simulink model "UberSpurs"  (R2015b)
settings: Solver=VariableStepAuto  StartTime=0.0  StopTime=5000  RelTol=1e-3
libraries: simulink x54
(part 2 of 6)

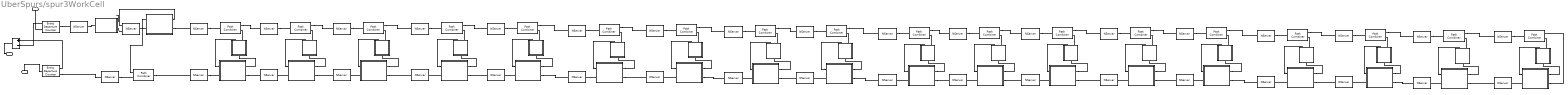
== system UberSpurs/spur3WorkCell ==
  Add1 : Sum  Inputs=+-
  INFlowCount : EntityDepartureCounter  NumberDepartedToSignal=on  NumberDepartedToAttribute=off
  OUTFlowCount : EntityDepartureCounter  NumberDepartedToSignal=on  NumberDepartedToAttribute=off
  combineRecirculate : PathCombiner  NumberInputPorts=2
  fillChannel1 : Subsystem
  fillChannel10 : Subsystem
  fillChannel11 : Subsystem
  fillChannel12 : Subsystem
  fillChannel13 : Subsystem
  fillChannel14 : Subsystem
  fillChannel15 : Subsystem
  fillChannel16 : Subsystem
  fillChannel17 : Subsystem
  fillChannel18 : Subsystem
  fillChannel2 : Subsystem
  fillChannel3 : Subsystem
  fillChannel4 : Subsystem
  fillChannel5 : Subsystem
  fillChannel6 : Subsystem
  fillChannel7 : Subsystem
  fillChannel8 : Subsystem
  fillChannel9 : Subsystem
  fromChannel{1..18} (18 alike) : PathCombiner  NumberInputPorts=2
  route2Channel1 : Subsystem
  route2Channel10 : Subsystem
  route2Channel11 : Subsystem
  route2Channel12 : Subsystem
  route2Channel13 : Subsystem
  route2Channel14 : Subsystem
  route2Channel15 : Subsystem
  route2Channel16 : Subsystem
  route2Channel17 : Subsystem
  route2Channel18 : Subsystem
  route2Channel2 : Subsystem
  route2Channel3 : Subsystem
  route2Channel4 : Subsystem
  route2Channel5 : Subsystem
  route2Channel6 : Subsystem
  route2Channel7 : Subsystem
  route2Channel8 : Subsystem
  route2Channel9 : Subsystem
  route2recirculate : Subsystem
  toChannel : NServer  NumberOfServers=15  ServiceTime=6
  toChannel{1..18} (18 alike) : NServer  NumberOfServers=2  ServiceTime=0.8
  toMainConveyor : NServer  ServiceTime=2
  toRecirculate : NServer  NumberOfServers=3
  toVerify : NServer  NumberOfServers=12  ServiceTime=5  StatNumberInBlock=on
      settings: OutputPortMap=o1
  toVerify{1..17} (17 alike) : NServer  NumberOfServers=2  ServiceTime=0.8
  verifyWorkstation : Subsystem
  toMHS : PMIOPort  Port=1  Side=Left
  fromMHS : PMIOPort  Port=2  Side=Left
  WIP : Outport
  wires:
  fillChannel1/1(serverAvailable) -> route2Channel1/1(serverAvailable)
  INFlowCount/1 -> Add1/1
  OUTFlowCount/1 -> Add1/2
  Add1/1 -> WIP/1
  fillChannel2/1(serverAvailable) -> route2Channel2/1(serverAvailable)
  fillChannel3/1(serverAvailable) -> route2Channel3/1(serverAvailable)
  fillChannel4/1(serverAvailable) -> route2Channel4/1(serverAvailable)
  fillChannel5/1(serverAvailable) -> route2Channel5/1(serverAvailable)
  fillChannel6/1(serverAvailable) -> route2Channel6/1(serverAvailable)
  fillChannel7/1(serverAvailable) -> route2Channel7/1(serverAvailable)
  fillChannel8/1(serverAvailable) -> route2Channel8/1(serverAvailable)
  fillChannel9/1(serverAvailable) -> route2Channel9/1(serverAvailable)
  fillChannel10/1(serverAvailable) -> route2Channel10/1(serverAvailable)
  fillChannel11/1(serverAvailable) -> route2Channel11/1(serverAvailable)
  fillChannel12/1(serverAvailable) -> route2Channel12/1(serverAvailable)
  fillChannel13/1(serverAvailable) -> route2Channel13/1(serverAvailable)
  fillChannel14/1(serverAvailable) -> route2Channel14/1(serverAvailable)
  fillChannel15/1(serverAvailable) -> route2Channel15/1(serverAvailable)
  fillChannel16/1(serverAvailable) -> route2Channel16/1(serverAvailable)
  fillChannel17/1(serverAvailable) -> route2Channel17/1(serverAvailable)
  fillChannel18/1(serverAvailable) -> route2Channel18/1(serverAvailable)
  toVerify/1 -> route2recirculate/1(verifyQueueLength)
  verifyWorkstation/1(queueLength) -> ?
  connections:
  fillChannel1/LConn1 -- route2Channel1/RConn1
  toChannel1/RConn1 -- route2Channel1/LConn1
  combineRecirculate/RConn1 -- toChannel1/LConn1
  route2recirculate/RConn1 -- combineRecirculate/LConn1
  OUTFlowCount/RConn1 -- toMHS/RConn1
  fromMHS/RConn1 -- INFlowCount/LConn1
  fillChannel1/RConn1 -- fromChannel1/LConn2
  toRecirculate/LConn1 -- fromChannel1/RConn1
  route2recirculate/LConn1 -- toRecirculate/RConn1
  route2Channel2/RConn1 -- fillChannel2/LConn1
  fillChannel2/RConn1 -- fromChannel2/LConn2
  route2Channel2/LConn1 -- toChannel2/RConn1
  toVerify1/LConn1 -- fromChannel2/RConn1
  route2Channel3/RConn1 -- fillChannel3/LConn1
  fillChannel3/RConn1 -- fromChannel3/LConn2
  route2Channel3/LConn1 -- toChannel3/RConn1
  toVerify2/LConn1 -- fromChannel3/RConn1
  route2Channel4/RConn1 -- fillChannel4/LConn1
  fillChannel4/RConn1 -- fromChannel4/LConn2
  route2Channel4/LConn1 -- toChannel4/RConn1
  toVerify3/LConn1 -- fromChannel4/RConn1
  route2Channel5/RConn1 -- fillChannel5/LConn1
  fillChannel5/RConn1 -- fromChannel5/LConn2
  route2Channel5/LConn1 -- toChannel5/RConn1
  toVerify4/LConn1 -- fromChannel5/RConn1
  route2Channel6/RConn1 -- fillChannel6/LConn1
  fillChannel6/RConn1 -- fromChannel6/LConn2
  route2Channel6/LConn1 -- toChannel6/RConn1
  toVerify5/LConn1 -- fromChannel6/RConn1
  route2Channel7/RConn1 -- fillChannel7/LConn1
  fillChannel7/RConn1 -- fromChannel7/LConn2
  route2Channel7/LConn1 -- toChannel7/RConn1
  toVerify6/LConn1 -- fromChannel7/RConn1
  route2Channel8/RConn1 -- fillChannel8/LConn1
  fillChannel8/RConn1 -- fromChannel8/LConn2
  route2Channel8/LConn1 -- toChannel8/RConn1
  toVerify7/LConn1 -- fromChannel8/RConn1
  route2Channel9/RConn1 -- fillChannel9/LConn1
  fillChannel9/RConn1 -- fromChannel9/LConn2
  route2Channel9/LConn1 -- toChannel9/RConn1
  toVerify8/LConn1 -- fromChannel9/RConn1
  fromChannel1/LConn1 -- toVerify1/RConn1
  route2Channel1/RConn2 -- toChannel2/LConn1
  route2Channel2/RConn2 -- toChannel3/LConn1
  fromChannel2/LConn1 -- toVerify2/RConn1
  fromChannel3/LConn1 -- toVerify3/RConn1
  route2Channel3/RConn2 -- toChannel4/LConn1
  fromChannel4/LConn1 -- toVerify4/RConn1
  route2Channel4/RConn2 -- toChannel5/LConn1
  fromChannel5/LConn1 -- toVerify5/RConn1
  route2Channel5/RConn2 -- toChannel6/LConn1
  fromChannel6/LConn1 -- toVerify6/RConn1
  route2Channel6/RConn2 -- toChannel7/LConn1
  fromChannel7/LConn1 -- toVerify7/RConn1
  route2Channel7/RConn2 -- toChannel8/LConn1
  fromChannel8/LConn1 -- toVerify8/RConn1
  route2Channel8/RConn2 -- toChannel9/LConn1
  route2Channel10/RConn2 -- toChannel11/LConn1
  route2Channel12/LConn1 -- toChannel12/RConn1
  route2Channel18/RConn1 -- fillChannel18/LConn1
  fromChannel17/LConn1 -- toVerify17/RConn1
  route2Channel13/RConn2 -- toChannel14/LConn1
  toVerify11/LConn1 -- fromChannel12/RConn1
  fillChannel10/RConn1 -- fromChannel10/LConn2
  fillChannel16/RConn1 -- fromChannel16/LConn2
  toVerify15/LConn1 -- fromChannel16/RConn1
  fromChannel14/LConn1 -- toVerify14/RConn1
  fillChannel15/RConn1 -- fromChannel15/LConn2
  toVerify14/LConn1 -- fromChannel15/RConn1
  route2Channel17/RConn2 -- toChannel18/LConn1
  fromChannel10/LConn1 -- toVerify10/RConn1
  toVerify17/LConn1 -- fromChannel18/RConn1
  route2Channel15/RConn2 -- toChannel16/LConn1
  route2Channel16/LConn1 -- toChannel16/RConn1
  route2Channel11/RConn2 -- toChannel12/LConn1
  toVerify9/LConn1 -- fromChannel10/RConn1
  route2Channel16/RConn2 -- toChannel17/LConn1
  fromChannel15/LConn1 -- toVerify15/RConn1
  toVerify12/LConn1 -- fromChannel13/RConn1
  route2Channel16/RConn1 -- fillChannel16/LConn1
  fromChannel13/LConn1 -- toVerify13/RConn1
  route2Channel15/RConn1 -- fillChannel15/LConn1
  fromChannel16/LConn1 -- toVerify16/RConn1
  route2Channel12/RConn1 -- fillChannel12/LConn1
  fillChannel18/RConn1 -- fromChannel18/LConn2
  route2Channel15/LConn1 -- toChannel15/RConn1
  route2Channel12/RConn2 -- toChannel13/LConn1
  route2Channel18/LConn1 -- toChannel18/RConn1
  fillChannel12/RConn1 -- fromChannel12/LConn2
  route2Channel14/RConn2 -- toChannel15/LConn1
  fromChannel11/LConn1 -- toVerify11/RConn1
  fromChannel12/LConn1 -- toVerify12/RConn1
  route2Channel13/LConn1 -- toChannel13/RConn1
  route2Channel10/LConn1 -- toChannel10/RConn1
  toVerify13/LConn1 -- fromChannel14/RConn1
  route2Channel17/RConn1 -- fillChannel17/LConn1
  fillChannel14/RConn1 -- fromChannel14/LConn2
  fillChannel11/RConn1 -- fromChannel11/LConn2
  route2Channel10/RConn1 -- fillChannel10/LConn1
  route2Channel11/LConn1 -- toChannel11/RConn1
  fillChannel17/RConn1 -- fromChannel17/LConn2
  route2Channel17/LConn1 -- toChannel17/RConn1
  route2Channel14/LConn1 -- toChannel14/RConn1
  toVerify16/LConn1 -- fromChannel17/RConn1
  route2Channel13/RConn1 -- fillChannel13/LConn1
  fillChannel13/RConn1 -- fromChannel13/LConn2
  route2Channel14/RConn1 -- fillChannel14/LConn1
  route2Channel11/RConn1 -- fillChannel11/LConn1
  toVerify10/LConn1 -- fromChannel11/RConn1
  fromChannel9/LConn1 -- toVerify9/RConn1
  route2Channel9/RConn2 -- toChannel10/LConn1
  route2Channel18/RConn2 -- fromChannel18/LConn1
  toChannel/RConn1 -- combineRecirculate/LConn2
  INFlowCount/RConn1 -- toChannel/LConn1
  toVerify/RConn1 -- verifyWorkstation/RConn1
  toVerify/LConn1 -- route2recirculate/RConn2
  toMainConveyor/LConn1 -- verifyWorkstation/LConn1
  OUTFlowCount/LConn1 -- toMainConveyor/RConn1

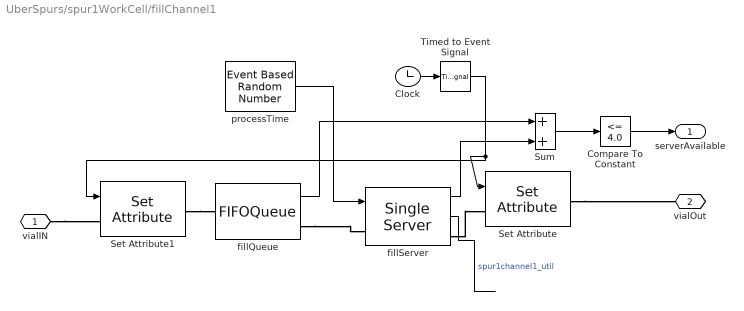
== system UberSpurs/spur1WorkCell/fillChannel1 ==
  Clock : Clock
  Compare To Constant : simulink/Logic and Bit Operations/Compare To Constant  relop=<=  const=4.0  OutDataTypeStr=boolean
  Set Attribute : SetAttribute  AttributeName=FillTime  AttributeFrom=Signal port  EvaluatedAttributeValue={ []}
  Set Attribute1 : SetAttribute  AttributeName=FillTimeIN  AttributeFrom=Signal port  EvaluatedAttributeValue={ []}
  Sum : Sum  Inputs=|++
  Timed to Event Signal : TimedToEventSignal
  fillQueue : FIFOQueue  Capacity=3  StatNumberInBlock=on
      settings: OutputPortMap=o1
  fillServer : SingleServer  ServiceTimeFrom=Signal port t  ServiceTime=20  StatNumberInBlock=on  StatUtilization=on
      settings: OutputPortMap=o1,o5
  processTime : EventBasedRandomNumber  Distribution=Gaussian (normal)  meanNorm=12  stdNorm=0.6  Seed=31208
  vialIN : PMIOPort  Port=1  Side=Left
  vialOut : PMIOPort  Port=2  Side=Right
  serverAvailable : Outport
  wires:
  processTime/1 -> fillServer/1
  Clock/1 -> Timed to Event Signal/1
  Timed to Event Signal/1 -> Set Attribute1/1, Set Attribute/1
  fillQueue/1 -> Sum/1
  fillServer/1 -> Sum/2
  Sum/1 -> Compare To Constant/1
  Compare To Constant/1 -> serverAvailable/1
  fillServer/2 -> ?  "spur1channel1_util"
  connections:
  fillQueue/RConn1 -- fillServer/LConn1
  fillServer/RConn1 -- Set Attribute/LConn1
  Set Attribute/RConn1 -- vialOut/RConn1
  vialIN/RConn1 -- Set Attribute1/LConn1
  Set Attribute1/RConn1 -- fillQueue/LConn1

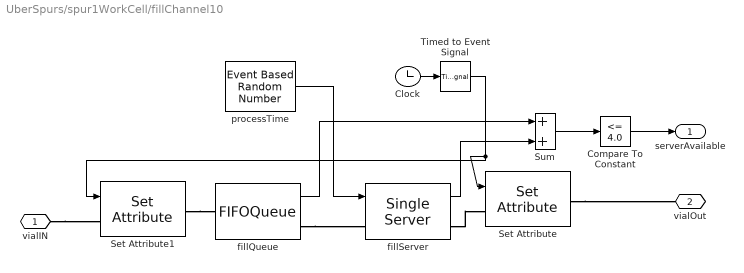
== system UberSpurs/spur1WorkCell/fillChannel10 ==
  Clock : Clock
  Compare To Constant : simulink/Logic and Bit Operations/Compare To Constant  relop=<=  const=4.0  OutDataTypeStr=boolean
  Set Attribute : SetAttribute  AttributeName=FillTime  AttributeFrom=Signal port  EvaluatedAttributeValue={ []}
  Set Attribute1 : SetAttribute  AttributeName=FillTimeIN  AttributeFrom=Signal port  EvaluatedAttributeValue={ []}
  Sum : Sum  Inputs=|++
  Timed to Event Signal : TimedToEventSignal
  fillQueue : FIFOQueue  Capacity=3  StatNumberInBlock=on
      settings: OutputPortMap=o1
  fillServer : SingleServer  ServiceTimeFrom=Signal port t  ServiceTime=20  StatNumberInBlock=on
      settings: OutputPortMap=o1
  processTime : EventBasedRandomNumber  Distribution=Gaussian (normal)  meanNorm=12  stdNorm=0.6  Seed=34425
  vialIN : PMIOPort  Port=1  Side=Left
  vialOut : PMIOPort  Port=2  Side=Right
  serverAvailable : Outport
  wires:
  processTime/1 -> fillServer/1
  Clock/1 -> Timed to Event Signal/1
  Timed to Event Signal/1 -> Set Attribute1/1, Set Attribute/1
  fillQueue/1 -> Sum/1
  fillServer/1 -> Sum/2
  Sum/1 -> Compare To Constant/1
  Compare To Constant/1 -> serverAvailable/1
  connections:
  fillQueue/RConn1 -- fillServer/LConn1
  fillServer/RConn1 -- Set Attribute/LConn1
  Set Attribute/RConn1 -- vialOut/RConn1
  vialIN/RConn1 -- Set Attribute1/LConn1
  Set Attribute1/RConn1 -- fillQueue/LConn1

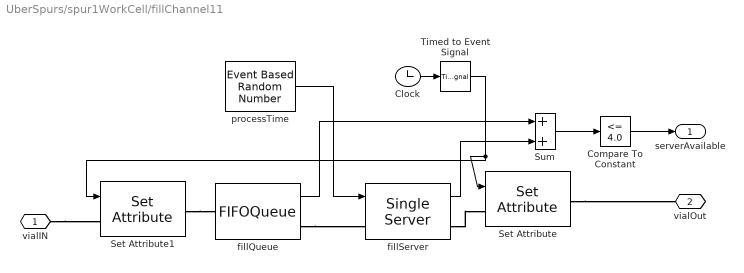
== system UberSpurs/spur1WorkCell/fillChannel11 ==
  Clock : Clock
  Compare To Constant : simulink/Logic and Bit Operations/Compare To Constant  relop=<=  const=4.0  OutDataTypeStr=boolean
  Set Attribute : SetAttribute  AttributeName=FillTime  AttributeFrom=Signal port  EvaluatedAttributeValue={ []}
  Set Attribute1 : SetAttribute  AttributeName=FillTimeIN  AttributeFrom=Signal port  EvaluatedAttributeValue={ []}
  Sum : Sum  Inputs=|++
  Timed to Event Signal : TimedToEventSignal
  fillQueue : FIFOQueue  Capacity=3  StatNumberInBlock=on
      settings: OutputPortMap=o1
  fillServer : SingleServer  ServiceTimeFrom=Signal port t  ServiceTime=20  StatNumberInBlock=on
      settings: OutputPortMap=o1
  processTime : EventBasedRandomNumber  Distribution=Gaussian (normal)  meanNorm=12  stdNorm=0.6  Seed=37642
  vialIN : PMIOPort  Port=1  Side=Left
  vialOut : PMIOPort  Port=2  Side=Right
  serverAvailable : Outport
  wires:
  processTime/1 -> fillServer/1
  Clock/1 -> Timed to Event Signal/1
  Timed to Event Signal/1 -> Set Attribute1/1, Set Attribute/1
  fillQueue/1 -> Sum/1
  fillServer/1 -> Sum/2
  Sum/1 -> Compare To Constant/1
  Compare To Constant/1 -> serverAvailable/1
  connections:
  fillQueue/RConn1 -- fillServer/LConn1
  fillServer/RConn1 -- Set Attribute/LConn1
  Set Attribute/RConn1 -- vialOut/RConn1
  vialIN/RConn1 -- Set Attribute1/LConn1
  Set Attribute1/RConn1 -- fillQueue/LConn1

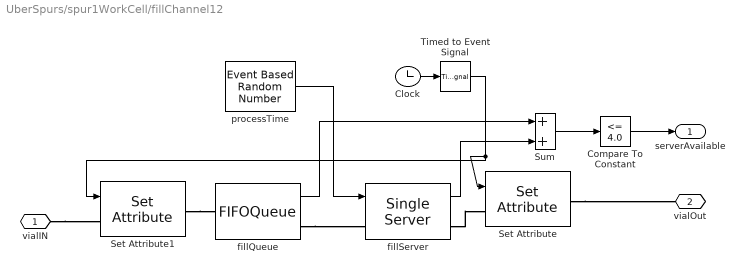
== system UberSpurs/spur1WorkCell/fillChannel12 ==
  Clock : Clock
  Compare To Constant : simulink/Logic and Bit Operations/Compare To Constant  relop=<=  const=4.0  OutDataTypeStr=boolean
  Set Attribute : SetAttribute  AttributeName=FillTime  AttributeFrom=Signal port  EvaluatedAttributeValue={ []}
  Set Attribute1 : SetAttribute  AttributeName=FillTimeIN  AttributeFrom=Signal port  EvaluatedAttributeValue={ []}
  Sum : Sum  Inputs=|++
  Timed to Event Signal : TimedToEventSignal
  fillQueue : FIFOQueue  Capacity=3  StatNumberInBlock=on
      settings: OutputPortMap=o1
  fillServer : SingleServer  ServiceTimeFrom=Signal port t  ServiceTime=20  StatNumberInBlock=on
      settings: OutputPortMap=o1
  processTime : EventBasedRandomNumber  Distribution=Gaussian (normal)  meanNorm=12  stdNorm=0.6  Seed=40859
  vialIN : PMIOPort  Port=1  Side=Left
  vialOut : PMIOPort  Port=2  Side=Right
  serverAvailable : Outport
  wires:
  processTime/1 -> fillServer/1
  Clock/1 -> Timed to Event Signal/1
  Timed to Event Signal/1 -> Set Attribute1/1, Set Attribute/1
  fillQueue/1 -> Sum/1
  fillServer/1 -> Sum/2
  Sum/1 -> Compare To Constant/1
  Compare To Constant/1 -> serverAvailable/1
  connections:
  fillQueue/RConn1 -- fillServer/LConn1
  fillServer/RConn1 -- Set Attribute/LConn1
  Set Attribute/RConn1 -- vialOut/RConn1
  vialIN/RConn1 -- Set Attribute1/LConn1
  Set Attribute1/RConn1 -- fillQueue/LConn1

== system UberSpurs/spur1WorkCell/fillChannel13 ==
  Clock : Clock
  Compare To Constant : simulink/Logic and Bit Operations/Compare To Constant  relop=<=  const=4.0  OutDataTypeStr=boolean
  Set Attribute : SetAttribute  AttributeName=FillTime  AttributeFrom=Signal port  EvaluatedAttributeValue={ []}
  Set Attribute1 : SetAttribute  AttributeName=FillTimeIN  AttributeFrom=Signal port  EvaluatedAttributeValue={ []}
  Sum : Sum  Inputs=|++
  Timed to Event Signal : TimedToEventSignal
  fillQueue : FIFOQueue  Capacity=3  StatNumberInBlock=on
      settings: OutputPortMap=o1
  fillServer : SingleServer  ServiceTimeFrom=Signal port t  ServiceTime=20  StatNumberInBlock=on
      settings: OutputPortMap=o1
  processTime : EventBasedRandomNumber  Distribution=Gaussian (normal)  meanNorm=12  stdNorm=0.6  Seed=44076
  vialIN : PMIOPort  Port=1  Side=Left
  vialOut : PMIOPort  Port=2  Side=Right
  serverAvailable : Outport
  wires:
  processTime/1 -> fillServer/1
  Clock/1 -> Timed to Event Signal/1
  Timed to Event Signal/1 -> Set Attribute1/1, Set Attribute/1
  fillQueue/1 -> Sum/1
  fillServer/1 -> Sum/2
  Sum/1 -> Compare To Constant/1
  Compare To Constant/1 -> serverAvailable/1
  connections:
  fillQueue/RConn1 -- fillServer/LConn1
  fillServer/RConn1 -- Set Attribute/LConn1
  Set Attribute/RConn1 -- vialOut/RConn1
  vialIN/RConn1 -- Set Attribute1/LConn1
  Set Attribute1/RConn1 -- fillQueue/LConn1

== system UberSpurs/spur1WorkCell/fillChannel14 ==
  Clock : Clock
  Compare To Constant : simulink/Logic and Bit Operations/Compare To Constant  relop=<=  const=4.0  OutDataTypeStr=boolean
  Set Attribute : SetAttribute  AttributeName=FillTime  AttributeFrom=Signal port  EvaluatedAttributeValue={ []}
  Set Attribute1 : SetAttribute  AttributeName=FillTimeIN  AttributeFrom=Signal port  EvaluatedAttributeValue={ []}
  Sum : Sum  Inputs=|++
  Timed to Event Signal : TimedToEventSignal
  fillQueue : FIFOQueue  Capacity=3  StatNumberInBlock=on
      settings: OutputPortMap=o1
  fillServer : SingleServer  ServiceTimeFrom=Signal port t  ServiceTime=20  StatNumberInBlock=on
      settings: OutputPortMap=o1
  processTime : EventBasedRandomNumber  Distribution=Gaussian (normal)  meanNorm=12  stdNorm=0.6  Seed=47293
  vialIN : PMIOPort  Port=1  Side=Left
  vialOut : PMIOPort  Port=2  Side=Right
  serverAvailable : Outport
  wires:
  processTime/1 -> fillServer/1
  Clock/1 -> Timed to Event Signal/1
  Timed to Event Signal/1 -> Set Attribute1/1, Set Attribute/1
  fillQueue/1 -> Sum/1
  fillServer/1 -> Sum/2
  Sum/1 -> Compare To Constant/1
  Compare To Constant/1 -> serverAvailable/1
  connections:
  fillQueue/RConn1 -- fillServer/LConn1
  fillServer/RConn1 -- Set Attribute/LConn1
  Set Attribute/RConn1 -- vialOut/RConn1
  vialIN/RConn1 -- Set Attribute1/LConn1
  Set Attribute1/RConn1 -- fillQueue/LConn1

== system UberSpurs/spur1WorkCell/fillChannel15 ==
  Clock : Clock
  Compare To Constant : simulink/Logic and Bit Operations/Compare To Constant  relop=<=  const=4.0  OutDataTypeStr=boolean
  Set Attribute : SetAttribute  AttributeName=FillTime  AttributeFrom=Signal port  EvaluatedAttributeValue={ []}
  Set Attribute1 : SetAttribute  AttributeName=FillTimeIN  AttributeFrom=Signal port  EvaluatedAttributeValue={ []}
  Sum : Sum  Inputs=|++
  Timed to Event Signal : TimedToEventSignal
  fillQueue : FIFOQueue  Capacity=3  StatNumberInBlock=on
      settings: OutputPortMap=o1
  fillServer : SingleServer  ServiceTimeFrom=Signal port t  ServiceTime=20  StatNumberInBlock=on
      settings: OutputPortMap=o1
  processTime : EventBasedRandomNumber  Distribution=Gaussian (normal)  meanNorm=12  stdNorm=0.6  Seed=50510
  vialIN : PMIOPort  Port=1  Side=Left
  vialOut : PMIOPort  Port=2  Side=Right
  serverAvailable : Outport
  wires:
  processTime/1 -> fillServer/1
  Clock/1 -> Timed to Event Signal/1
  Timed to Event Signal/1 -> Set Attribute1/1, Set Attribute/1
  fillQueue/1 -> Sum/1
  fillServer/1 -> Sum/2
  Sum/1 -> Compare To Constant/1
  Compare To Constant/1 -> serverAvailable/1
  connections:
  fillQueue/RConn1 -- fillServer/LConn1
  fillServer/RConn1 -- Set Attribute/LConn1
  Set Attribute/RConn1 -- vialOut/RConn1
  vialIN/RConn1 -- Set Attribute1/LConn1
  Set Attribute1/RConn1 -- fillQueue/LConn1

== system UberSpurs/spur1WorkCell/fillChannel16 ==
  Clock : Clock
  Compare To Constant : simulink/Logic and Bit Operations/Compare To Constant  relop=<=  const=4.0  OutDataTypeStr=boolean
  Set Attribute : SetAttribute  AttributeName=FillTime  AttributeFrom=Signal port  EvaluatedAttributeValue={ []}
  Set Attribute1 : SetAttribute  AttributeName=FillTimeIN  AttributeFrom=Signal port  EvaluatedAttributeValue={ []}
  Sum : Sum  Inputs=|++
  Timed to Event Signal : TimedToEventSignal
  fillQueue : FIFOQueue  Capacity=3  StatNumberInBlock=on
      settings: OutputPortMap=o1
  fillServer : SingleServer  ServiceTimeFrom=Signal port t  ServiceTime=20  StatNumberInBlock=on
      settings: OutputPortMap=o1
  processTime : EventBasedRandomNumber  Distribution=Gaussian (normal)  meanNorm=12  stdNorm=0.6  Seed=53727
  vialIN : PMIOPort  Port=1  Side=Left
  vialOut : PMIOPort  Port=2  Side=Right
  serverAvailable : Outport
  wires:
  processTime/1 -> fillServer/1
  Clock/1 -> Timed to Event Signal/1
  Timed to Event Signal/1 -> Set Attribute1/1, Set Attribute/1
  fillQueue/1 -> Sum/1
  fillServer/1 -> Sum/2
  Sum/1 -> Compare To Constant/1
  Compare To Constant/1 -> serverAvailable/1
  connections:
  fillQueue/RConn1 -- fillServer/LConn1
  fillServer/RConn1 -- Set Attribute/LConn1
  Set Attribute/RConn1 -- vialOut/RConn1
  vialIN/RConn1 -- Set Attribute1/LConn1
  Set Attribute1/RConn1 -- fillQueue/LConn1

== system UberSpurs/spur1WorkCell/fillChannel17 ==
  Clock : Clock
  Compare To Constant : simulink/Logic and Bit Operations/Compare To Constant  relop=<=  const=4.0  OutDataTypeStr=boolean
  Set Attribute : SetAttribute  AttributeName=FillTime  AttributeFrom=Signal port  EvaluatedAttributeValue={ []}
  Set Attribute1 : SetAttribute  AttributeName=FillTimeIN  AttributeFrom=Signal port  EvaluatedAttributeValue={ []}
  Sum : Sum  Inputs=|++
  Timed to Event Signal : TimedToEventSignal
  fillQueue : FIFOQueue  Capacity=3  StatNumberInBlock=on
      settings: OutputPortMap=o1
  fillServer : SingleServer  ServiceTimeFrom=Signal port t  ServiceTime=20  StatNumberInBlock=on
      settings: OutputPortMap=o1
  processTime : EventBasedRandomNumber  Distribution=Gaussian (normal)  meanNorm=12  stdNorm=0.6  Seed=56944
  vialIN : PMIOPort  Port=1  Side=Left
  vialOut : PMIOPort  Port=2  Side=Right
  serverAvailable : Outport
  wires:
  processTime/1 -> fillServer/1
  Clock/1 -> Timed to Event Signal/1
  Timed to Event Signal/1 -> Set Attribute1/1, Set Attribute/1
  fillQueue/1 -> Sum/1
  fillServer/1 -> Sum/2
  Sum/1 -> Compare To Constant/1
  Compare To Constant/1 -> serverAvailable/1
  connections:
  fillQueue/RConn1 -- fillServer/LConn1
  fillServer/RConn1 -- Set Attribute/LConn1
  Set Attribute/RConn1 -- vialOut/RConn1
  vialIN/RConn1 -- Set Attribute1/LConn1
  Set Attribute1/RConn1 -- fillQueue/LConn1

== system UberSpurs/spur1WorkCell/fillChannel18 ==
  Clock : Clock
  Compare To Constant : simulink/Logic and Bit Operations/Compare To Constant  relop=<=  const=4.0  OutDataTypeStr=boolean
  Set Attribute : SetAttribute  AttributeName=FillTime  AttributeFrom=Signal port  EvaluatedAttributeValue={ []}
  Set Attribute1 : SetAttribute  AttributeName=FillTimeIN  AttributeFrom=Signal port  EvaluatedAttributeValue={ []}
  Sum : Sum  Inputs=|++
  Timed to Event Signal : TimedToEventSignal
  fillQueue : FIFOQueue  Capacity=3  StatNumberInBlock=on
      settings: OutputPortMap=o1
  fillServer : SingleServer  ServiceTimeFrom=Signal port t  ServiceTime=20  StatNumberInBlock=on
      settings: OutputPortMap=o1
  processTime : EventBasedRandomNumber  Distribution=Gaussian (normal)  meanNorm=12  stdNorm=0.6  Seed=60161
  vialIN : PMIOPort  Port=1  Side=Left
  vialOut : PMIOPort  Port=2  Side=Right
  serverAvailable : Outport
  wires:
  processTime/1 -> fillServer/1
  Clock/1 -> Timed to Event Signal/1
  Timed to Event Signal/1 -> Set Attribute1/1, Set Attribute/1
  fillQueue/1 -> Sum/1
  fillServer/1 -> Sum/2
  Sum/1 -> Compare To Constant/1
  Compare To Constant/1 -> serverAvailable/1
  connections:
  fillQueue/RConn1 -- fillServer/LConn1
  fillServer/RConn1 -- Set Attribute/LConn1
  Set Attribute/RConn1 -- vialOut/RConn1
  vialIN/RConn1 -- Set Attribute1/LConn1
  Set Attribute1/RConn1 -- fillQueue/LConn1

== system UberSpurs/spur1WorkCell/fillChannel2 ==
  Clock : Clock
  Compare To Constant : simulink/Logic and Bit Operations/Compare To Constant  relop=<=  const=4.0  OutDataTypeStr=boolean
  Set Attribute : SetAttribute  AttributeName=FillTime  AttributeFrom=Signal port  EvaluatedAttributeValue={ []}
  Set Attribute1 : SetAttribute  AttributeName=FillTimeIN  AttributeFrom=Signal port  EvaluatedAttributeValue={ []}
  Sum : Sum  Inputs=|++
  Timed to Event Signal : TimedToEventSignal
  fillQueue : FIFOQueue  Capacity=3  StatNumberInBlock=on
      settings: OutputPortMap=o1
  fillServer : SingleServer  ServiceTimeFrom=Signal port t  ServiceTime=20  StatNumberInBlock=on
      settings: OutputPortMap=o1
  processTime : EventBasedRandomNumber  Distribution=Gaussian (normal)  meanNorm=12  stdNorm=0.6  Seed=63378
  vialIN : PMIOPort  Port=1  Side=Left
  vialOut : PMIOPort  Port=2  Side=Right
  serverAvailable : Outport
  wires:
  processTime/1 -> fillServer/1
  Clock/1 -> Timed to Event Signal/1
  Timed to Event Signal/1 -> Set Attribute1/1, Set Attribute/1
  fillQueue/1 -> Sum/1
  fillServer/1 -> Sum/2
  Sum/1 -> Compare To Constant/1
  Compare To Constant/1 -> serverAvailable/1
  connections:
  fillQueue/RConn1 -- fillServer/LConn1
  fillServer/RConn1 -- Set Attribute/LConn1
  Set Attribute/RConn1 -- vialOut/RConn1
  vialIN/RConn1 -- Set Attribute1/LConn1
  Set Attribute1/RConn1 -- fillQueue/LConn1

== system UberSpurs/spur1WorkCell/fillChannel3 ==
  Clock : Clock
  Compare To Constant : simulink/Logic and Bit Operations/Compare To Constant  relop=<=  const=4.0  OutDataTypeStr=boolean
  Set Attribute : SetAttribute  AttributeName=FillTime  AttributeFrom=Signal port  EvaluatedAttributeValue={ []}
  Set Attribute1 : SetAttribute  AttributeName=FillTimeIN  AttributeFrom=Signal port  EvaluatedAttributeValue={ []}
  Sum : Sum  Inputs=|++
  Timed to Event Signal : TimedToEventSignal
  fillQueue : FIFOQueue  Capacity=3  StatNumberInBlock=on
      settings: OutputPortMap=o1
  fillServer : SingleServer  ServiceTimeFrom=Signal port t  ServiceTime=20  StatNumberInBlock=on
      settings: OutputPortMap=o1
  processTime : EventBasedRandomNumber  Distribution=Gaussian (normal)  meanNorm=12  stdNorm=0.6  Seed=1059
  vialIN : PMIOPort  Port=1  Side=Left
  vialOut : PMIOPort  Port=2  Side=Right
  serverAvailable : Outport
  wires:
  processTime/1 -> fillServer/1
  Clock/1 -> Timed to Event Signal/1
  Timed to Event Signal/1 -> Set Attribute1/1, Set Attribute/1
  fillQueue/1 -> Sum/1
  fillServer/1 -> Sum/2
  Sum/1 -> Compare To Constant/1
  Compare To Constant/1 -> serverAvailable/1
  connections:
  fillQueue/RConn1 -- fillServer/LConn1
  fillServer/RConn1 -- Set Attribute/LConn1
  Set Attribute/RConn1 -- vialOut/RConn1
  vialIN/RConn1 -- Set Attribute1/LConn1
  Set Attribute1/RConn1 -- fillQueue/LConn1

== system UberSpurs/spur1WorkCell/fillChannel4 ==
  Clock : Clock
  Compare To Constant : simulink/Logic and Bit Operations/Compare To Constant  relop=<=  const=4.0  OutDataTypeStr=boolean
  Set Attribute : SetAttribute  AttributeName=FillTime  AttributeFrom=Signal port  EvaluatedAttributeValue={ []}
  Set Attribute1 : SetAttribute  AttributeName=FillTimeIN  AttributeFrom=Signal port  EvaluatedAttributeValue={ []}
  Sum : Sum  Inputs=|++
  Timed to Event Signal : TimedToEventSignal
  fillQueue : FIFOQueue  Capacity=3  StatNumberInBlock=on
      settings: OutputPortMap=o1
  fillServer : SingleServer  ServiceTimeFrom=Signal port t  ServiceTime=20  StatNumberInBlock=on
      settings: OutputPortMap=o1
  processTime : EventBasedRandomNumber  Distribution=Gaussian (normal)  meanNorm=12  stdNorm=0.6  Seed=4276
  vialIN : PMIOPort  Port=1  Side=Left
  vialOut : PMIOPort  Port=2  Side=Right
  serverAvailable : Outport
  wires:
  processTime/1 -> fillServer/1
  Clock/1 -> Timed to Event Signal/1
  Timed to Event Signal/1 -> Set Attribute1/1, Set Attribute/1
  fillQueue/1 -> Sum/1
  fillServer/1 -> Sum/2
  Sum/1 -> Compare To Constant/1
  Compare To Constant/1 -> serverAvailable/1
  connections:
  fillQueue/RConn1 -- fillServer/LConn1
  fillServer/RConn1 -- Set Attribute/LConn1
  Set Attribute/RConn1 -- vialOut/RConn1
  vialIN/RConn1 -- Set Attribute1/LConn1
  Set Attribute1/RConn1 -- fillQueue/LConn1

== system UberSpurs/spur1WorkCell/fillChannel5 ==
  Clock : Clock
  Compare To Constant : simulink/Logic and Bit Operations/Compare To Constant  relop=<=  const=4.0  OutDataTypeStr=boolean
  Set Attribute : SetAttribute  AttributeName=FillTime  AttributeFrom=Signal port  EvaluatedAttributeValue={ []}
  Set Attribute1 : SetAttribute  AttributeName=FillTimeIN  AttributeFrom=Signal port  EvaluatedAttributeValue={ []}
  Sum : Sum  Inputs=|++
  Timed to Event Signal : TimedToEventSignal
  fillQueue : FIFOQueue  Capacity=3  StatNumberInBlock=on
      settings: OutputPortMap=o1
  fillServer : SingleServer  ServiceTimeFrom=Signal port t  ServiceTime=20  StatNumberInBlock=on
      settings: OutputPortMap=o1
  processTime : EventBasedRandomNumber  Distribution=Gaussian (normal)  meanNorm=12  stdNorm=0.6  Seed=7493
  vialIN : PMIOPort  Port=1  Side=Left
  vialOut : PMIOPort  Port=2  Side=Right
  serverAvailable : Outport
  wires:
  processTime/1 -> fillServer/1
  Clock/1 -> Timed to Event Signal/1
  Timed to Event Signal/1 -> Set Attribute1/1, Set Attribute/1
  fillQueue/1 -> Sum/1
  fillServer/1 -> Sum/2
  Sum/1 -> Compare To Constant/1
  Compare To Constant/1 -> serverAvailable/1
  connections:
  fillQueue/RConn1 -- fillServer/LConn1
  fillServer/RConn1 -- Set Attribute/LConn1
  Set Attribute/RConn1 -- vialOut/RConn1
  vialIN/RConn1 -- Set Attribute1/LConn1
  Set Attribute1/RConn1 -- fillQueue/LConn1

== system UberSpurs/spur1WorkCell/fillChannel6 ==
  Clock : Clock
  Compare To Constant : simulink/Logic and Bit Operations/Compare To Constant  relop=<=  const=4.0  OutDataTypeStr=boolean
  Set Attribute : SetAttribute  AttributeName=FillTime  AttributeFrom=Signal port  EvaluatedAttributeValue={ []}
  Set Attribute1 : SetAttribute  AttributeName=FillTimeIN  AttributeFrom=Signal port  EvaluatedAttributeValue={ []}
  Sum : Sum  Inputs=|++
  Timed to Event Signal : TimedToEventSignal
  fillQueue : FIFOQueue  Capacity=3  StatNumberInBlock=on
      settings: OutputPortMap=o1
  fillServer : SingleServer  ServiceTimeFrom=Signal port t  ServiceTime=20  StatNumberInBlock=on
      settings: OutputPortMap=o1
  processTime : EventBasedRandomNumber  Distribution=Gaussian (normal)  meanNorm=12  stdNorm=0.6  Seed=10710
  vialIN : PMIOPort  Port=1  Side=Left
  vialOut : PMIOPort  Port=2  Side=Right
  serverAvailable : Outport
  wires:
  processTime/1 -> fillServer/1
  Clock/1 -> Timed to Event Signal/1
  Timed to Event Signal/1 -> Set Attribute1/1, Set Attribute/1
  fillQueue/1 -> Sum/1
  fillServer/1 -> Sum/2
  Sum/1 -> Compare To Constant/1
  Compare To Constant/1 -> serverAvailable/1
  connections:
  fillQueue/RConn1 -- fillServer/LConn1
  fillServer/RConn1 -- Set Attribute/LConn1
  Set Attribute/RConn1 -- vialOut/RConn1
  vialIN/RConn1 -- Set Attribute1/LConn1
  Set Attribute1/RConn1 -- fillQueue/LConn1

== system UberSpurs/spur1WorkCell/fillChannel7 ==
  Clock : Clock
  Compare To Constant : simulink/Logic and Bit Operations/Compare To Constant  relop=<=  const=4.0  OutDataTypeStr=boolean
  Set Attribute : SetAttribute  AttributeName=FillTime  AttributeFrom=Signal port  EvaluatedAttributeValue={ []}
  Set Attribute1 : SetAttribute  AttributeName=FillTimeIN  AttributeFrom=Signal port  EvaluatedAttributeValue={ []}
  Sum : Sum  Inputs=|++
  Timed to Event Signal : TimedToEventSignal
  fillQueue : FIFOQueue  Capacity=3  StatNumberInBlock=on
      settings: OutputPortMap=o1
  fillServer : SingleServer  ServiceTimeFrom=Signal port t  ServiceTime=20  StatNumberInBlock=on
      settings: OutputPortMap=o1
  processTime : EventBasedRandomNumber  Distribution=Gaussian (normal)  meanNorm=12  stdNorm=0.6  Seed=13927
  vialIN : PMIOPort  Port=1  Side=Left
  vialOut : PMIOPort  Port=2  Side=Right
  serverAvailable : Outport
  wires:
  processTime/1 -> fillServer/1
  Clock/1 -> Timed to Event Signal/1
  Timed to Event Signal/1 -> Set Attribute1/1, Set Attribute/1
  fillQueue/1 -> Sum/1
  fillServer/1 -> Sum/2
  Sum/1 -> Compare To Constant/1
  Compare To Constant/1 -> serverAvailable/1
  connections:
  fillQueue/RConn1 -- fillServer/LConn1
  fillServer/RConn1 -- Set Attribute/LConn1
  Set Attribute/RConn1 -- vialOut/RConn1
  vialIN/RConn1 -- Set Attribute1/LConn1
  Set Attribute1/RConn1 -- fillQueue/LConn1

== system UberSpurs/spur1WorkCell/fillChannel8 ==
  Clock : Clock
  Compare To Constant : simulink/Logic and Bit Operations/Compare To Constant  relop=<=  const=4.0  OutDataTypeStr=boolean
  Set Attribute : SetAttribute  AttributeName=FillTime  AttributeFrom=Signal port  EvaluatedAttributeValue={ []}
  Set Attribute1 : SetAttribute  AttributeName=FillTimeIN  AttributeFrom=Signal port  EvaluatedAttributeValue={ []}
  Sum : Sum  Inputs=|++
  Timed to Event Signal : TimedToEventSignal
  fillQueue : FIFOQueue  Capacity=3  StatNumberInBlock=on
      settings: OutputPortMap=o1
  fillServer : SingleServer  ServiceTimeFrom=Signal port t  ServiceTime=20  StatNumberInBlock=on
      settings: OutputPortMap=o1
  processTime : EventBasedRandomNumber  Distribution=Gaussian (normal)  meanNorm=12  stdNorm=0.6  Seed=17144
  vialIN : PMIOPort  Port=1  Side=Left
  vialOut : PMIOPort  Port=2  Side=Right
  serverAvailable : Outport
  wires:
  processTime/1 -> fillServer/1
  Clock/1 -> Timed to Event Signal/1
  Timed to Event Signal/1 -> Set Attribute1/1, Set Attribute/1
  fillQueue/1 -> Sum/1
  fillServer/1 -> Sum/2
  Sum/1 -> Compare To Constant/1
  Compare To Constant/1 -> serverAvailable/1
  connections:
  fillQueue/RConn1 -- fillServer/LConn1
  fillServer/RConn1 -- Set Attribute/LConn1
  Set Attribute/RConn1 -- vialOut/RConn1
  vialIN/RConn1 -- Set Attribute1/LConn1
  Set Attribute1/RConn1 -- fillQueue/LConn1

== system UberSpurs/spur1WorkCell/fillChannel9 ==
  Clock : Clock
  Compare To Constant : simulink/Logic and Bit Operations/Compare To Constant  relop=<=  const=4.0  OutDataTypeStr=boolean
  Set Attribute : SetAttribute  AttributeName=FillTime  AttributeFrom=Signal port  EvaluatedAttributeValue={ []}
  Set Attribute1 : SetAttribute  AttributeName=FillTimeIN  AttributeFrom=Signal port  EvaluatedAttributeValue={ []}
  Sum : Sum  Inputs=|++
  Timed to Event Signal : TimedToEventSignal
  fillQueue : FIFOQueue  Capacity=3  StatNumberInBlock=on
      settings: OutputPortMap=o1
  fillServer : SingleServer  ServiceTimeFrom=Signal port t  ServiceTime=20  StatNumberInBlock=on
      settings: OutputPortMap=o1
  processTime : EventBasedRandomNumber  Distribution=Gaussian (normal)  meanNorm=12  stdNorm=0.6  Seed=20361
  vialIN : PMIOPort  Port=1  Side=Left
  vialOut : PMIOPort  Port=2  Side=Right
  serverAvailable : Outport
  wires:
  processTime/1 -> fillServer/1
  Clock/1 -> Timed to Event Signal/1
  Timed to Event Signal/1 -> Set Attribute1/1, Set Attribute/1
  fillQueue/1 -> Sum/1
  fillServer/1 -> Sum/2
  Sum/1 -> Compare To Constant/1
  Compare To Constant/1 -> serverAvailable/1
  connections:
  fillQueue/RConn1 -- fillServer/LConn1
  fillServer/RConn1 -- Set Attribute/LConn1
  Set Attribute/RConn1 -- vialOut/RConn1
  vialIN/RConn1 -- Set Attribute1/LConn1
  Set Attribute1/RConn1 -- fillQueue/LConn1

== system UberSpurs/spur1WorkCell/route2Channel1 ==
  serverAvailable : Inport
  Constant : Constant
  Get Attribute : GetAttribute  AttributeName=Channel|FillTime  AttributeMissing=Error|Error  AttributeDefaultValue=1|1  AttributeTreatAsVector=1|1  AttributeSendTiming=After entity departure|After entity departure  EvaluatedDefaultAttributeValue={ [];[]}
      settings: OutputPortMap=o1,o2
  RoutingControlActuator : OutputSwitch  NumberOutputPorts=2  SwitchingCriterion=From signal port p  InitialConditionsOpt=on
  RoutingControlBehavior : Stateflow chart  TreatAsAtomicUnit=on
  Single Server1 : SingleServer  ServiceTime=0
  toChannel : PMIOPort  Port=1  Side=Right
  fromMHS : PMIOPort  Port=2  Side=Left
  toMHS : PMIOPort  Port=3  Side=Right
  wires:
  RoutingControlBehavior/1(route) -> RoutingControlActuator/1
  Constant/1 -> RoutingControlBehavior/2(channel)
  Get Attribute/1 -> RoutingControlBehavior/1(entityChannel)
  serverAvailable/1 -> RoutingControlBehavior/3(serverAvailable)
  Get Attribute/2 -> RoutingControlBehavior/4(FillTime)
  connections:
  RoutingControlActuator/RConn2 -- toMHS/RConn1
  Get Attribute/RConn1 -- Single Server1/LConn1
  fromMHS/RConn1 -- Get Attribute/LConn1
  toChannel/RConn1 -- RoutingControlActuator/RConn1
  Single Server1/RConn1 -- RoutingControlActuator/LConn1

== system UberSpurs/spur1WorkCell/route2Channel10 ==
  serverAvailable : Inport
  Constant : Constant  Value=10
  Get Attribute : GetAttribute  AttributeName=Channel|FillTime  AttributeMissing=Error|Error  AttributeDefaultValue=1|1  AttributeTreatAsVector=1|1  AttributeSendTiming=After entity departure|After entity departure  EvaluatedDefaultAttributeValue={ [];[]}
      settings: OutputPortMap=o1,o2
  RoutingControlActuator : OutputSwitch  NumberOutputPorts=2  SwitchingCriterion=From signal port p  InitialConditionsOpt=on
  RoutingControlBehavior : Stateflow chart  TreatAsAtomicUnit=on
  Single Server1 : SingleServer  ServiceTime=0
  toChannel : PMIOPort  Port=1  Side=Right
  fromMHS : PMIOPort  Port=2  Side=Left
  toMHS : PMIOPort  Port=3  Side=Right
  wires:
  RoutingControlBehavior/1(route) -> RoutingControlActuator/1
  Constant/1 -> RoutingControlBehavior/2(channel)
  Get Attribute/1 -> RoutingControlBehavior/1(entityChannel)
  serverAvailable/1 -> RoutingControlBehavior/3(serverAvailable)
  Get Attribute/2 -> RoutingControlBehavior/4(FillTime)
  connections:
  RoutingControlActuator/RConn2 -- toMHS/RConn1
  Get Attribute/RConn1 -- Single Server1/LConn1
  fromMHS/RConn1 -- Get Attribute/LConn1
  toChannel/RConn1 -- RoutingControlActuator/RConn1
  Single Server1/RConn1 -- RoutingControlActuator/LConn1

== system UberSpurs/spur1WorkCell/route2Channel11 ==
  serverAvailable : Inport
  Constant : Constant  Value=11
  Get Attribute : GetAttribute  AttributeName=Channel|FillTime  AttributeMissing=Error|Error  AttributeDefaultValue=1|1  AttributeTreatAsVector=1|1  AttributeSendTiming=After entity departure|After entity departure  EvaluatedDefaultAttributeValue={ [];[]}
      settings: OutputPortMap=o1,o2
  RoutingControlActuator : OutputSwitch  NumberOutputPorts=2  SwitchingCriterion=From signal port p  InitialConditionsOpt=on
  RoutingControlBehavior : Stateflow chart  TreatAsAtomicUnit=on
  Single Server1 : SingleServer  ServiceTime=0
  toChannel : PMIOPort  Port=1  Side=Right
  fromMHS : PMIOPort  Port=2  Side=Left
  toMHS : PMIOPort  Port=3  Side=Right
  wires:
  RoutingControlBehavior/1(route) -> RoutingControlActuator/1
  Constant/1 -> RoutingControlBehavior/2(channel)
  Get Attribute/1 -> RoutingControlBehavior/1(entityChannel)
  serverAvailable/1 -> RoutingControlBehavior/3(serverAvailable)
  Get Attribute/2 -> RoutingControlBehavior/4(FillTime)
  connections:
  RoutingControlActuator/RConn2 -- toMHS/RConn1
  Get Attribute/RConn1 -- Single Server1/LConn1
  fromMHS/RConn1 -- Get Attribute/LConn1
  toChannel/RConn1 -- RoutingControlActuator/RConn1
  Single Server1/RConn1 -- RoutingControlActuator/LConn1

== system UberSpurs/spur1WorkCell/route2Channel12 ==
  serverAvailable : Inport
  Constant : Constant  Value=12
  Get Attribute : GetAttribute  AttributeName=Channel|FillTime  AttributeMissing=Error|Error  AttributeDefaultValue=1|1  AttributeTreatAsVector=1|1  AttributeSendTiming=After entity departure|After entity departure  EvaluatedDefaultAttributeValue={ [];[]}
      settings: OutputPortMap=o1,o2
  RoutingControlActuator : OutputSwitch  NumberOutputPorts=2  SwitchingCriterion=From signal port p  InitialConditionsOpt=on
  RoutingControlBehavior : Stateflow chart  TreatAsAtomicUnit=on
  Single Server1 : SingleServer  ServiceTime=0
  toChannel : PMIOPort  Port=1  Side=Right
  fromMHS : PMIOPort  Port=2  Side=Left
  toMHS : PMIOPort  Port=3  Side=Right
  wires:
  RoutingControlBehavior/1(route) -> RoutingControlActuator/1
  Constant/1 -> RoutingControlBehavior/2(channel)
  Get Attribute/1 -> RoutingControlBehavior/1(entityChannel)
  serverAvailable/1 -> RoutingControlBehavior/3(serverAvailable)
  Get Attribute/2 -> RoutingControlBehavior/4(FillTime)
  connections:
  RoutingControlActuator/RConn2 -- toMHS/RConn1
  Get Attribute/RConn1 -- Single Server1/LConn1
  fromMHS/RConn1 -- Get Attribute/LConn1
  toChannel/RConn1 -- RoutingControlActuator/RConn1
  Single Server1/RConn1 -- RoutingControlActuator/LConn1

== system UberSpurs/spur1WorkCell/route2Channel13 ==
  serverAvailable : Inport
  Constant : Constant  Value=13
  Get Attribute : GetAttribute  AttributeName=Channel|FillTime  AttributeMissing=Error|Error  AttributeDefaultValue=1|1  AttributeTreatAsVector=1|1  AttributeSendTiming=After entity departure|After entity departure  EvaluatedDefaultAttributeValue={ [];[]}
      settings: OutputPortMap=o1,o2
  RoutingControlActuator : OutputSwitch  NumberOutputPorts=2  SwitchingCriterion=From signal port p  InitialConditionsOpt=on
  RoutingControlBehavior : Stateflow chart  TreatAsAtomicUnit=on
  Single Server1 : SingleServer  ServiceTime=0
  toChannel : PMIOPort  Port=1  Side=Right
  fromMHS : PMIOPort  Port=2  Side=Left
  toMHS : PMIOPort  Port=3  Side=Right
  wires:
  RoutingControlBehavior/1(route) -> RoutingControlActuator/1
  Constant/1 -> RoutingControlBehavior/2(channel)
  Get Attribute/1 -> RoutingControlBehavior/1(entityChannel)
  serverAvailable/1 -> RoutingControlBehavior/3(serverAvailable)
  Get Attribute/2 -> RoutingControlBehavior/4(FillTime)
  connections:
  RoutingControlActuator/RConn2 -- toMHS/RConn1
  Get Attribute/RConn1 -- Single Server1/LConn1
  fromMHS/RConn1 -- Get Attribute/LConn1
  toChannel/RConn1 -- RoutingControlActuator/RConn1
  Single Server1/RConn1 -- RoutingControlActuator/LConn1

== system UberSpurs/spur1WorkCell/route2Channel14 ==
  serverAvailable : Inport
  Constant : Constant  Value=14
  Get Attribute : GetAttribute  AttributeName=Channel|FillTime  AttributeMissing=Error|Error  AttributeDefaultValue=1|1  AttributeTreatAsVector=1|1  AttributeSendTiming=After entity departure|After entity departure  EvaluatedDefaultAttributeValue={ [];[]}
      settings: OutputPortMap=o1,o2
  RoutingControlActuator : OutputSwitch  NumberOutputPorts=2  SwitchingCriterion=From signal port p  InitialConditionsOpt=on
  RoutingControlBehavior : Stateflow chart  TreatAsAtomicUnit=on
  Single Server1 : SingleServer  ServiceTime=0
  toChannel : PMIOPort  Port=1  Side=Right
  fromMHS : PMIOPort  Port=2  Side=Left
  toMHS : PMIOPort  Port=3  Side=Right
  wires:
  RoutingControlBehavior/1(route) -> RoutingControlActuator/1
  Constant/1 -> RoutingControlBehavior/2(channel)
  Get Attribute/1 -> RoutingControlBehavior/1(entityChannel)
  serverAvailable/1 -> RoutingControlBehavior/3(serverAvailable)
  Get Attribute/2 -> RoutingControlBehavior/4(FillTime)
  connections:
  RoutingControlActuator/RConn2 -- toMHS/RConn1
  Get Attribute/RConn1 -- Single Server1/LConn1
  fromMHS/RConn1 -- Get Attribute/LConn1
  toChannel/RConn1 -- RoutingControlActuator/RConn1
  Single Server1/RConn1 -- RoutingControlActuator/LConn1

== system UberSpurs/spur1WorkCell/route2Channel15 ==
  serverAvailable : Inport
  Constant : Constant  Value=15
  Get Attribute : GetAttribute  AttributeName=Channel|FillTime  AttributeMissing=Error|Error  AttributeDefaultValue=1|1  AttributeTreatAsVector=1|1  AttributeSendTiming=After entity departure|After entity departure  EvaluatedDefaultAttributeValue={ [];[]}
      settings: OutputPortMap=o1,o2
  RoutingControlActuator : OutputSwitch  NumberOutputPorts=2  SwitchingCriterion=From signal port p  InitialConditionsOpt=on
  RoutingControlBehavior : Stateflow chart  TreatAsAtomicUnit=on
  Single Server1 : SingleServer  ServiceTime=0
  toChannel : PMIOPort  Port=1  Side=Right
  fromMHS : PMIOPort  Port=2  Side=Left
  toMHS : PMIOPort  Port=3  Side=Right
  wires:
  RoutingControlBehavior/1(route) -> RoutingControlActuator/1
  Constant/1 -> RoutingControlBehavior/2(channel)
  Get Attribute/1 -> RoutingControlBehavior/1(entityChannel)
  serverAvailable/1 -> RoutingControlBehavior/3(serverAvailable)
  Get Attribute/2 -> RoutingControlBehavior/4(FillTime)
  connections:
  RoutingControlActuator/RConn2 -- toMHS/RConn1
  Get Attribute/RConn1 -- Single Server1/LConn1
  fromMHS/RConn1 -- Get Attribute/LConn1
  toChannel/RConn1 -- RoutingControlActuator/RConn1
  Single Server1/RConn1 -- RoutingControlActuator/LConn1

== system UberSpurs/spur1WorkCell/route2Channel16 ==
  serverAvailable : Inport
  Constant : Constant  Value=16
  Get Attribute : GetAttribute  AttributeName=Channel|FillTime  AttributeMissing=Error|Error  AttributeDefaultValue=1|1  AttributeTreatAsVector=1|1  AttributeSendTiming=After entity departure|After entity departure  EvaluatedDefaultAttributeValue={ [];[]}
      settings: OutputPortMap=o1,o2
  RoutingControlActuator : OutputSwitch  NumberOutputPorts=2  SwitchingCriterion=From signal port p  InitialConditionsOpt=on
  RoutingControlBehavior : Stateflow chart  TreatAsAtomicUnit=on
  Single Server1 : SingleServer  ServiceTime=0
  toChannel : PMIOPort  Port=1  Side=Right
  fromMHS : PMIOPort  Port=2  Side=Left
  toMHS : PMIOPort  Port=3  Side=Right
  wires:
  RoutingControlBehavior/1(route) -> RoutingControlActuator/1
  Constant/1 -> RoutingControlBehavior/2(channel)
  Get Attribute/1 -> RoutingControlBehavior/1(entityChannel)
  serverAvailable/1 -> RoutingControlBehavior/3(serverAvailable)
  Get Attribute/2 -> RoutingControlBehavior/4(FillTime)
  connections:
  RoutingControlActuator/RConn2 -- toMHS/RConn1
  Get Attribute/RConn1 -- Single Server1/LConn1
  fromMHS/RConn1 -- Get Attribute/LConn1
  toChannel/RConn1 -- RoutingControlActuator/RConn1
  Single Server1/RConn1 -- RoutingControlActuator/LConn1

== system UberSpurs/spur1WorkCell/route2Channel17 ==
  serverAvailable : Inport
  Constant : Constant  Value=17
  Get Attribute : GetAttribute  AttributeName=Channel|FillTime  AttributeMissing=Error|Error  AttributeDefaultValue=1|1  AttributeTreatAsVector=1|1  AttributeSendTiming=After entity departure|After entity departure  EvaluatedDefaultAttributeValue={ [];[]}
      settings: OutputPortMap=o1,o2
  RoutingControlActuator : OutputSwitch  NumberOutputPorts=2  SwitchingCriterion=From signal port p  InitialConditionsOpt=on
  RoutingControlBehavior : Stateflow chart  TreatAsAtomicUnit=on
  Single Server1 : SingleServer  ServiceTime=0
  toChannel : PMIOPort  Port=1  Side=Right
  fromMHS : PMIOPort  Port=2  Side=Left
  toMHS : PMIOPort  Port=3  Side=Right
  wires:
  RoutingControlBehavior/1(route) -> RoutingControlActuator/1
  Constant/1 -> RoutingControlBehavior/2(channel)
  Get Attribute/1 -> RoutingControlBehavior/1(entityChannel)
  serverAvailable/1 -> RoutingControlBehavior/3(serverAvailable)
  Get Attribute/2 -> RoutingControlBehavior/4(FillTime)
  connections:
  RoutingControlActuator/RConn2 -- toMHS/RConn1
  Get Attribute/RConn1 -- Single Server1/LConn1
  fromMHS/RConn1 -- Get Attribute/LConn1
  toChannel/RConn1 -- RoutingControlActuator/RConn1
  Single Server1/RConn1 -- RoutingControlActuator/LConn1

== system UberSpurs/spur1WorkCell/route2Channel18 ==
  serverAvailable : Inport
  Constant : Constant  Value=18
  Get Attribute : GetAttribute  AttributeName=Channel|FillTime  AttributeMissing=Error|Error  AttributeDefaultValue=1|1  AttributeTreatAsVector=1|1  AttributeSendTiming=After entity departure|After entity departure  EvaluatedDefaultAttributeValue={ [];[]}
      settings: OutputPortMap=o1,o2
  RoutingControlActuator : OutputSwitch  NumberOutputPorts=2  SwitchingCriterion=From signal port p  InitialConditionsOpt=on
  RoutingControlBehavior : Stateflow chart  TreatAsAtomicUnit=on
  Single Server1 : SingleServer  ServiceTime=0
  toChannel : PMIOPort  Port=1  Side=Right
  fromMHS : PMIOPort  Port=2  Side=Left
  toMHS : PMIOPort  Port=3  Side=Right
  wires:
  RoutingControlBehavior/1(route) -> RoutingControlActuator/1
  Constant/1 -> RoutingControlBehavior/2(channel)
  Get Attribute/1 -> RoutingControlBehavior/1(entityChannel)
  serverAvailable/1 -> RoutingControlBehavior/3(serverAvailable)
  Get Attribute/2 -> RoutingControlBehavior/4(FillTime)
  connections:
  RoutingControlActuator/RConn2 -- toMHS/RConn1
  Get Attribute/RConn1 -- Single Server1/LConn1
  fromMHS/RConn1 -- Get Attribute/LConn1
  toChannel/RConn1 -- RoutingControlActuator/RConn1
  Single Server1/RConn1 -- RoutingControlActuator/LConn1

== system UberSpurs/spur1WorkCell/route2Channel2 ==
  serverAvailable : Inport
  Constant : Constant  Value=2
  Get Attribute : GetAttribute  AttributeName=Channel|FillTime  AttributeMissing=Error|Error  AttributeDefaultValue=1|1  AttributeTreatAsVector=1|1  AttributeSendTiming=After entity departure|After entity departure  EvaluatedDefaultAttributeValue={ [];[]}
      settings: OutputPortMap=o1,o2
  RoutingControlActuator : OutputSwitch  NumberOutputPorts=2  SwitchingCriterion=From signal port p  InitialConditionsOpt=on
  RoutingControlBehavior : Stateflow chart  TreatAsAtomicUnit=on
  Single Server1 : SingleServer  ServiceTime=0
  toChannel : PMIOPort  Port=1  Side=Right
  fromMHS : PMIOPort  Port=2  Side=Left
  toMHS : PMIOPort  Port=3  Side=Right
  wires:
  RoutingControlBehavior/1(route) -> RoutingControlActuator/1
  Constant/1 -> RoutingControlBehavior/2(channel)
  Get Attribute/1 -> RoutingControlBehavior/1(entityChannel)
  serverAvailable/1 -> RoutingControlBehavior/3(serverAvailable)
  Get Attribute/2 -> RoutingControlBehavior/4(FillTime)
  connections:
  RoutingControlActuator/RConn2 -- toMHS/RConn1
  Get Attribute/RConn1 -- Single Server1/LConn1
  fromMHS/RConn1 -- Get Attribute/LConn1
  toChannel/RConn1 -- RoutingControlActuator/RConn1
  Single Server1/RConn1 -- RoutingControlActuator/LConn1
